simulink model "test"  (Simulink 9.0)
settings: Solver=VariableStepAuto  StartTime=0.0  StopTime=20  FixedStep=0.001  RelTol=1e-3
libraries: Solver_SF x1, simulink x1
settings Model: Creator=zhang  LastModifiedBy=zhang
settings DataIOCC: SaveFormat=Dataset
settings OptimizationCC: LifeSpan=auto
settings DebuggingCC: UnderspecifiedInitializationDetection=Simplified  MergeDetectMultiDrivingBlocksExec=error  SFUnexpectedBacktrackingDiag=error  SFNoUnconditionalDefaultTransitionDiag=error  SFExecutionAtInitializationDiag=warning
settings HardwareCC: ProdBitPerPointer=64  ProdBitPerSizeT=64  ProdBitPerPtrDiffT=64  ProdLargestAtomicFloat=Float  ProdIntDivRoundTo=Zero  ProdEndianess=LittleEndian  ProdWordSize=64  ProdHWDeviceType=Intel->x86-64 (Windows64)
settings ModelReferenceCC: PropagateSignalLabelsOutOfModel=on
settings CodeAppCC: StateflowObjectComments=off
settings GRTTargetCC: TargetLangStandard=C99 (ISO)
settings ConfigComp: CovMetricSettings=dwe  CovHtmlReporting=off  CovSaveCumulativeToWorkspaceVar=off  CovSaveSingleToWorkspaceVar=off  CovExternalEMLEnable=on

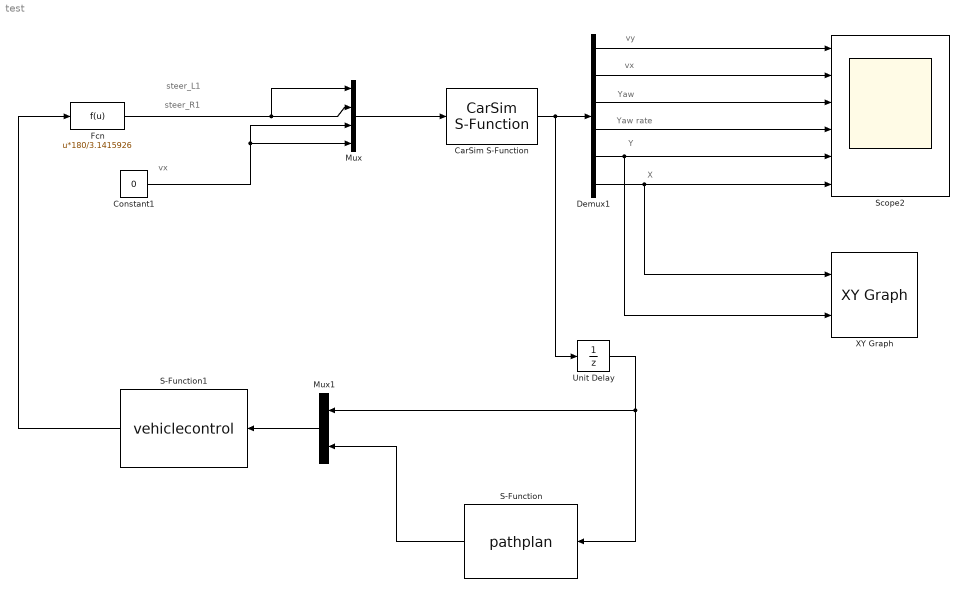
== system test ==
  note: X
  note: Y
  note: Yaw rate
  note: Yaw
  note: vx
  note: vy
  note: vx
  note: steer_R1
  note: steer_L1
  CarSim S-Function : Solver_SF/CarSim S-Function  Priority=1  VehicleCode=i_i  SIMFILE=simfile.sim
  Constant1 : Constant  Value=0
  Demux1 : Demux  Outputs=6
  Fcn : Fcn  Expr=u*180/3.1415926
  Mux : Mux
  Mux1 : Mux  Inputs=2
  S-Function : S-Function  FunctionName=pathplan  SFunctionDeploymentMode=off  EnableBusSupport=off
  S-Function1 : S-Function  FunctionName=vehiclecontrol  SFunctionDeploymentMode=off  EnableBusSupport=off
  Scope2 : Scope  NumInputPorts=6
  Unit Delay : UnitDelay  InitialCondition=[0 36 0 0 0 0]  SampleTime=-1
  XY Graph : simulink/Sinks/XY Graph  xmin=0  xmax=250  ymin=-3  ymax=6  st=-1
  wires:
  Mux/1 -> CarSim S-Function/1
  Fcn/1 -> Mux/1, Mux/2
  CarSim S-Function/1 -> Unit Delay/1, Demux1/1
  Demux1/1 -> Scope2/1
  Demux1/2 -> Scope2/2
  Demux1/3 -> Scope2/3
  Demux1/4 -> Scope2/4
  Demux1/5 -> XY Graph/2, Scope2/5
  Demux1/6 -> XY Graph/1, Scope2/6
  Constant1/1 -> Mux/4, Mux/3
  Unit Delay/1 -> Mux1/1, S-Function/1
  S-Function/1 -> Mux1/2
  Mux1/1 -> S-Function1/1
  S-Function1/1 -> Fcn/1
